simulink model "SS_discreto"  (R2022b)
settings: Solver=VariableStepAuto  StartTime=0.0  StopTime=10.0  RelTol=1e-3
values from neighbouring files (symbols this model uses):
  rpm2rads = 2*pi/60    (= 0.10471975512)    [load_params_inertial_case.m]
undefined symbols (not defined in the file or in its folder): aw_sw, DiscIntNeverNeededParam, H_0, int, J_0, Kw, nom, Nu, Nx, phi_0, rho_0, sens, T
settings Model: Creator=marcoverri  LastModifiedBy=marcoverri

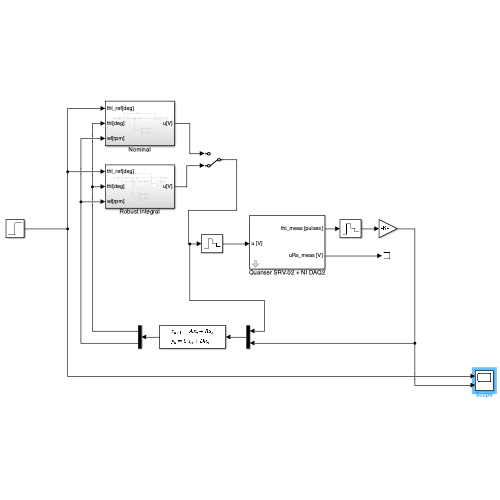
[thumbnail: Simulink's stored preview of the top-level diagram]
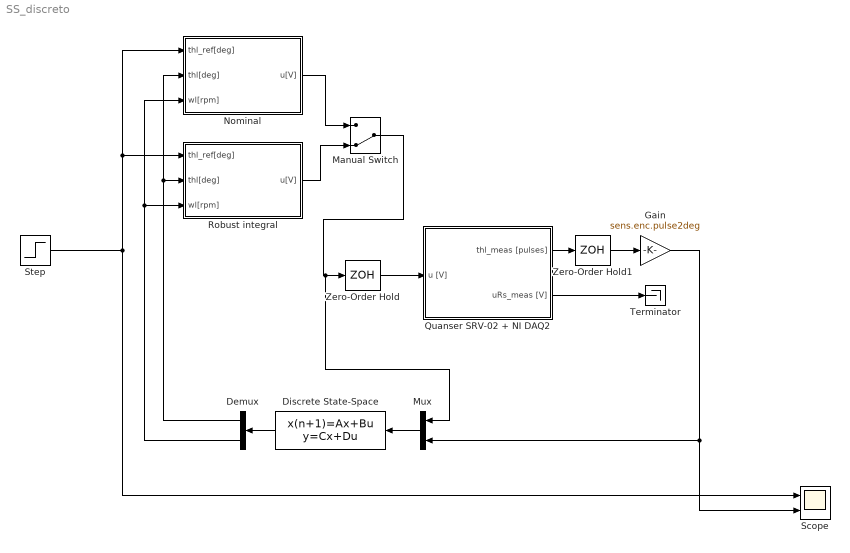
== system SS_discreto ==
  Demux : Demux  Outputs=2
  Discrete State-Space : DiscreteStateSpace  A=phi_0  B=rho_0  C=H_0  D=J_0  SampleTime=T
  Gain : Gain  Gain=sens.enc.pulse2deg
  Manual Switch : ManualSwitch  CurrentSetting=0
  Mux : Mux  Inputs=2
  Nominal : Subsystem
  Quanser SRV-02 + NI DAQ2 : Subsystem  mask(Quanser SRV-02 (with inertial load) + NI DAQ){Ts=0.001, fricType=Coulomb + viscous}
      mask prompts: Ts "NI DAQ Sample Time:"; fricType "Friction model"
      mask help: Quanser SRV-02 (with inertial load) + NI DAQ model.
      mask init:
      | %%  Sensors data
      | 
      | %   shunt resistor
      | sens.curr.Rs = 0.5;                         %   resistance [Ohm]   
      | sens.curr.uRs_std = 0.01;                   %   voltage noise standard dev [V]                           
      | sens.curr.uRs_var = sens.curr.uRs_std^2;	%   voltage noise variance [V^2]
      | 
      | %   Hewlett-Packard HEDS-5540#A06 optical encoder
      | sens.enc.ppr = 500*4;                       %   pulses per rotation
      | sens.enc.pulse2deg = 360/sens.enc.ppr;      %   [pulses] -> [deg]
      | sens.enc.pulse2rad = 2*pi/sens.enc.ppr;     %   [pulses] -> [rad]
      | sens.enc.deg2pulse = sens.enc.ppr/360;      %   [deg] -> [pulses]
      | sens.enc.rad2pulse = sens.enc.ppr/2/pi;     %   [rad] -> [pulses]
      | 
      | 
      | %%  Data acquisition board (daq) data
      | 
      | %   NI PCI-6221 DAC data
      | daq.dac.bits = 16;                                  %   resolution (bits)
      | daq.dac.fs   = 10;                                  %   full scale 
      | daq.dac.q    = 2*daq.dac.fs/(2^daq.dac.bits-1);     %	quantization
      | 
      | %   NI PCI-6221 ADC data
      | daq.adc.bits = 16;                                  %   resolution (bits)
      | daq.adc.fs   = 10;                                  %   full scale (as set in SLDRT Analog Input block)
      | daq.adc.q    = 2*daq.adc.fs/(2^daq.adc.bits-1);     %   quantization
      mask Help:
      | Riccardo Antonello (antonello@dei.unipd.it)
      | 
      | April 24, 2020
      | 
      | Dept. of Information Engineering, University of Padova
      mask TypeOptions fricType: Coulomb + viscous | Karnopp
  Robust integral : Subsystem
  Scope : Scope  NumInputPorts=2
  Step : Step  After=50  SampleTime=0
  Terminator : Terminator
  Zero-Order Hold : ZeroOrderHold  SampleTime=-1
  Zero-Order Hold1 : ZeroOrderHold  SampleTime=-1
  wires:
  Demux/2 -> Robust integral/3(wl[rpm]), Nominal/3(wl[rpm])
  Quanser SRV-02 + NI DAQ2/1(thl_meas [pulses]) -> Zero-Order Hold1/1
  Quanser SRV-02 + NI DAQ2/2(uRs_meas [V]) -> Terminator/1
  Demux/1 -> Robust integral/2(thl[deg]), Nominal/2(thl[deg])
  Step/1 -> Scope/1, Robust integral/1(thl_ref[deg]), Nominal/1(thl_ref[deg])
  Gain/1 -> Mux/2, Scope/2
  Zero-Order Hold/1 -> Quanser SRV-02 + NI DAQ2/1(u [V])
  Zero-Order Hold1/1 -> Gain/1
  Mux/1 -> Discrete State-Space/1
  Discrete State-Space/1 -> Demux/1
  Robust integral/1(u[V]) -> Manual Switch/2
  Nominal/1(u[V]) -> Manual Switch/1
  Manual Switch/1 -> Mux/1, Zero-Order Hold/1

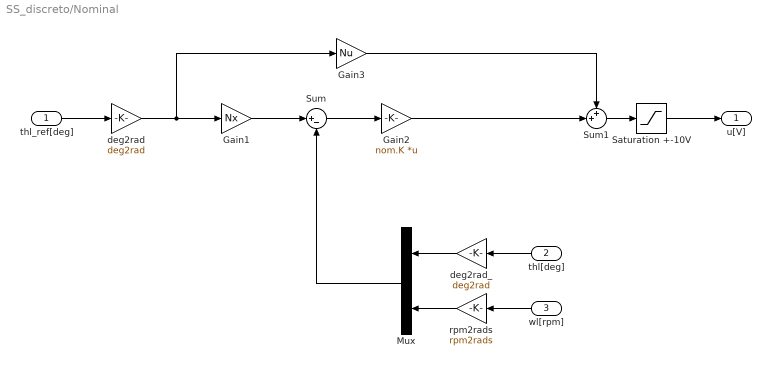
== system SS_discreto/Nominal ==
  thl_ref[deg] : Inport
  thl[deg] : Inport  Port=2
  wl[rpm] : Inport  Port=3
  Gain1 : Gain  Gain=Nx
  Gain2 : Gain  Gain=nom.K  Multiplication=Matrix(K*u)
  Gain3 : Gain  Gain=Nu
  Mux : Mux  Inputs=2
  Saturation +-10V : Saturate  UpperLimit=10  LowerLimit=-10
  Sum : Sum  Inputs=|+-
  Sum1 : Sum  Inputs=++|
  deg2rad : Gain  Gain=deg2rad
  deg2rad_ : Gain  Gain=deg2rad
  rpm2rads : Gain  Gain=rpm2rads
  u[V] : Outport
  wires:
  thl_ref[deg]/1 -> deg2rad/1
  deg2rad/1 -> Gain3/1, Gain1/1
  Gain1/1 -> Sum/1
  Sum/1 -> Gain2/1
  Gain2/1 -> Sum1/2
  Gain3/1 -> Sum1/1
  Sum1/1 -> Saturation +-10V/1
  Saturation +-10V/1 -> u[V]/1
  Mux/1 -> Sum/2
  deg2rad_/1 -> Mux/1
  thl[deg]/1 -> deg2rad_/1
  wl[rpm]/1 -> rpm2rads/1
  rpm2rads/1 -> Mux/2

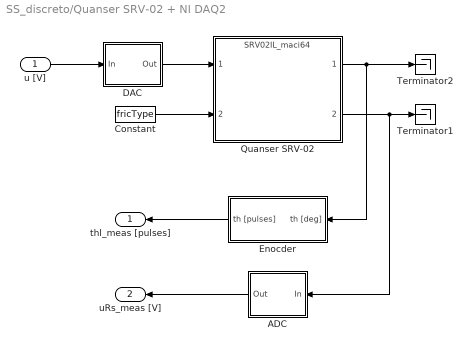
== system SS_discreto/Quanser SRV-02 + NI DAQ2 ==
  u [V] : Inport
  ADC : Subsystem
  Constant : Constant  Value=fricType
  DAC : Subsystem
  Enocder : Subsystem
  Quanser SRV-02 : ModelReference  ModelNameDialog=SRV02IL_maci64.slxp  ModelReferenceVersion=1.44  CopyOfModelProtected=on
  Terminator1 : Terminator
  Terminator2 : Terminator
  thl_meas [pulses] : Outport
  uRs_meas [V] : Outport  Port=2
  wires:
  Enocder/1(th [pulses]) -> thl_meas [pulses]/1
  ADC/1(Out) -> uRs_meas [V]/1
  DAC/1(Out) -> Quanser SRV-02/1
  Quanser SRV-02/2 -> ADC/1(In), Terminator1/1
  u [V]/1 -> DAC/1(In)
  Quanser SRV-02/1 -> Enocder/1(th [deg]), Terminator2/1
  Constant/1 -> Quanser SRV-02/2

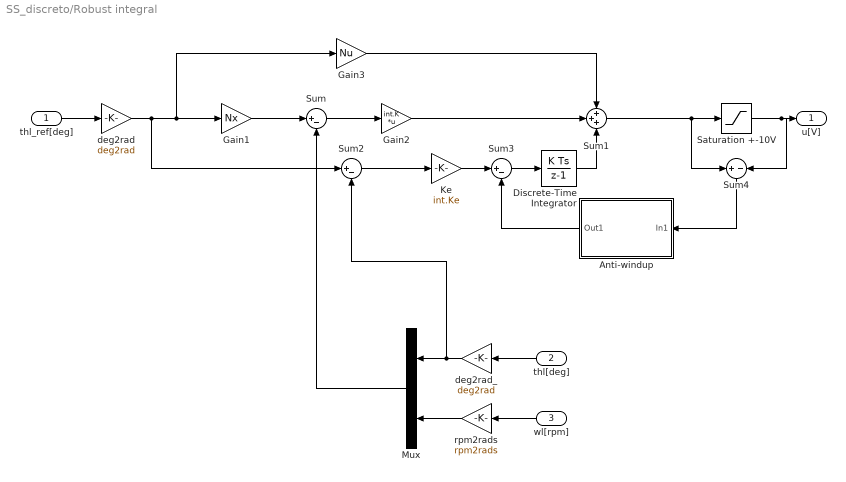
== system SS_discreto/Robust integral ==
  thl_ref[deg] : Inport
  thl[deg] : Inport  Port=2
  wl[rpm] : Inport  Port=3
  Anti-windup : Subsystem
  Discrete-Time Integrator : DiscreteIntegrator  SampleTime=-1  ICPrevOutput=DiscIntNeverNeededParam  ICPrevScaledInput=DiscIntNeverNeededParam
  Gain1 : Gain  Gain=Nx
  Gain2 : Gain  Gain=int.K  Multiplication=Matrix(K*u)
  Gain3 : Gain  Gain=Nu
  Ke : Gain  Gain=int.Ke
  Mux : Mux  Inputs=2
  Saturation +-10V : Saturate  UpperLimit=10  LowerLimit=-10
  Sum : Sum  Inputs=|+-
  Sum1 : Sum  Inputs=+++
  Sum2 : Sum  Inputs=|+-
  Sum3 : Sum  Inputs=|+-
  Sum4 : Sum  Inputs=+|-
  deg2rad : Gain  Gain=deg2rad
  deg2rad_ : Gain  Gain=deg2rad
  rpm2rads : Gain  Gain=rpm2rads
  u[V] : Outport
  wires:
  wl[rpm]/1 -> rpm2rads/1
  thl[deg]/1 -> deg2rad_/1
  Gain3/1 -> Sum1/1
  rpm2rads/1 -> Mux/2
  thl_ref[deg]/1 -> deg2rad/1
  Gain2/1 -> Sum1/2
  Mux/1 -> Sum/2
  Gain1/1 -> Sum/1
  deg2rad_/1 -> Sum2/2, Mux/1
  deg2rad/1 -> Sum2/1, Gain3/1, Gain1/1
  Sum/1 -> Gain2/1
  Sum2/1 -> Ke/1
  Discrete-Time Integrator/1 -> Sum1/3
  Saturation +-10V/1 -> Sum4/2, u[V]/1
  Sum1/1 -> Sum4/1, Saturation +-10V/1
  Anti-windup/1(Out1) -> Sum3/2
  Sum4/1 -> Anti-windup/1(In1)
  Ke/1 -> Sum3/1
  Sum3/1 -> Discrete-Time Integrator/1

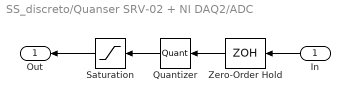
== system SS_discreto/Quanser SRV-02 + NI DAQ2/ADC ==
  In : Inport
  Quantizer : Quantizer  QuantizationInterval=daq.adc.q
  Saturation : Saturate  UpperLimit=daq.adc.fs  LowerLimit=-daq.adc.fs
  Zero-Order Hold : ZeroOrderHold  SampleTime=Ts
  Out : Outport
  wires:
  Saturation/1 -> Out/1
  In/1 -> Zero-Order Hold/1
  Quantizer/1 -> Saturation/1
  Zero-Order Hold/1 -> Quantizer/1

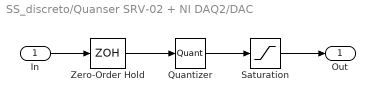
== system SS_discreto/Quanser SRV-02 + NI DAQ2/DAC ==
  In : Inport
  Quantizer : Quantizer  QuantizationInterval=daq.dac.q
  Saturation : Saturate  UpperLimit=daq.dac.fs  LowerLimit=-daq.dac.fs
  Zero-Order Hold : ZeroOrderHold  SampleTime=Ts
  Out : Outport
  wires:
  Quantizer/1 -> Saturation/1
  In/1 -> Zero-Order Hold/1
  Zero-Order Hold/1 -> Quantizer/1
  Saturation/1 -> Out/1

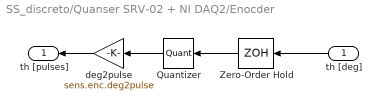
== system SS_discreto/Quanser SRV-02 + NI DAQ2/Enocder ==
  th [deg] : Inport
  Quantizer : Quantizer  QuantizationInterval=sens.enc.pulse2deg
  Zero-Order Hold : ZeroOrderHold  SampleTime=Ts
  deg2pulse : Gain  Gain=sens.enc.deg2pulse
  th [pulses] : Outport
  wires:
  Quantizer/1 -> deg2pulse/1
  th [deg]/1 -> Zero-Order Hold/1
  Zero-Order Hold/1 -> Quantizer/1
  deg2pulse/1 -> th [pulses]/1

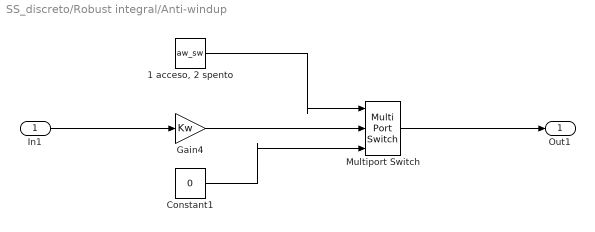
== system SS_discreto/Robust integral/Anti-windup ==
  In1 : Inport
  "1 acceso, 2 spento" : Constant  Value=aw_sw
  Constant1 : Constant  Value=0
  Gain4 : Gain  Gain=Kw
  Multiport Switch : MultiPortSwitch  Inputs=2  SaturateOnIntegerOverflow=off  InputSameDT=off
  Out1 : Outport
  wires:
  Multiport Switch/1 -> Out1/1
  In1/1 -> Gain4/1
  Gain4/1 -> Multiport Switch/2
  "1 acceso, 2 spento"/1 -> Multiport Switch/1
  Constant1/1 -> Multiport Switch/3
